simulink model "controllerSoln"  (R2018a)
settings: Solver=FixedStepAuto  StartTime=0.0  StopTime=10.0  RelTol=1e-3
PreLoadFcn:
  | initParams;
undefined symbols (not defined in the file or in its folder): DiscIntNeverNeededParam, Fc, Kd, Ki, Kp, Ts
settings Model: TunableVars=Kd,Ki,Kp  TunableVarsStorageClass=ExportedGlobal,ExportedGlobal,ExportedGlobal  TunableVarsTypeQualifier=,,  Creator=sseshadr  LastModifiedBy=scastro
settings DataIOCC: ExternalInput=testData1  LoadExternalInput=on  SaveFormat=Array
settings OptimizationCC: DefaultParameterBehavior=Inlined  EnhancedBackFolding=on  GlobalBufferReuse=off  PassReuseOutputArgsAs=Individual arguments  ZeroExternalMemoryAtStartup=off  ZeroInternalMemoryAtStartup=off  OptimizeBlockOrder=speed  DifferentSizesBufferReuse=on
settings DebuggingCC: ParameterTunabilityLossMsg=error
settings SFSimCC: MATLABDynamicMemAlloc=off
settings RTWCC: SystemTargetFile=ert.tlc  TemplateMakefile=ert_default_tmf  GenerateReport=on  IncludeHyperlinkInReport=on  LaunchReport=on  GenerateTraceInfo=on  GenerateTraceReport=on  GenerateTraceReportSl=on  GenerateTraceReportSf=on  GenerateTraceReportEml=on
settings CodeAppCC: ForceParamTrailComments=on  IgnoreCustomStorageClasses=off  OperatorAnnotations=on  SimulinkDataObjDesc=on  SFDataObjDesc=on  InsertBlockDesc=on
settings ERTTargetCC: TargetLangStandard=C99 (ISO)  GenerateSampleERTMain=on  IncludeMdlTerminateFcn=off  MatFileLogging=on  SupportComplex=off  InlinedParameterPlacement=NonHierarchical  ERTCustomFileTemplate=example_file_process.tlc

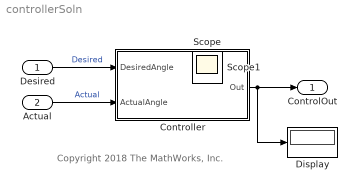
== system controllerSoln ==
  note: Copyright 2018 The MathWorks, Inc.
  Desired : Inport
  Actual : Inport  Port=2
  Controller : Subsystem
  Display : Display
  ControlOut : Outport
  Scope : Scope
  Scope1 : Scope
  wires:
  Controller/1(Out) -> Display/1, ControlOut/1
  Desired/1 -> Controller/1(DesiredAngle)  "Desired"
  Actual/1 -> Controller/2(ActualAngle)  "Actual"

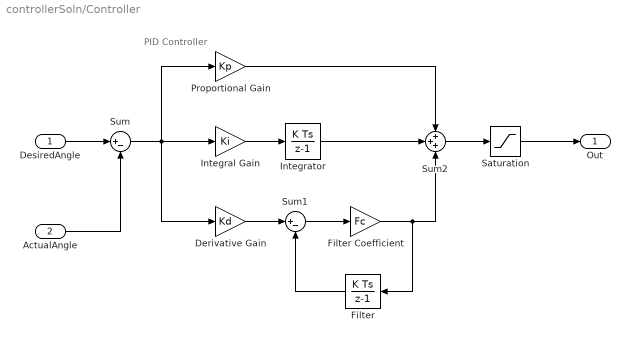
== system controllerSoln/Controller ==
  note: PID Controller
  DesiredAngle : Inport
  ActualAngle : Inport  Port=2
  Derivative Gain : Gain  Gain=Kd
  Filter : DiscreteIntegrator  DisableCoverage=on  SampleTime=Ts  ICPrevOutput=DiscIntNeverNeededParam  ICPrevScaledInput=DiscIntNeverNeededParam
  Filter Coefficient : Gain  Gain=Fc
  Integral Gain : Gain  Gain=Ki
  Integrator : DiscreteIntegrator  SampleTime=Ts  ICPrevOutput=DiscIntNeverNeededParam  ICPrevScaledInput=DiscIntNeverNeededParam
  Proportional Gain : Gain  Gain=Kp
  Saturation : Saturate  UpperLimit=5  LowerLimit=-5
  Sum : Sum  Inputs=|+-
  Sum1 : Sum  Inputs=|+-
  Sum2 : Sum  Inputs=+++
  Out : Outport
  wires:
  ActualAngle/1 -> Sum/2
  DesiredAngle/1 -> Sum/1
  Saturation/1 -> Out/1
  Sum/1 -> Derivative Gain/1, Proportional Gain/1, Integral Gain/1
  Integral Gain/1 -> Integrator/1
  Derivative Gain/1 -> Sum1/1
  Filter/1 -> Sum1/2
  Sum1/1 -> Filter Coefficient/1
  Filter Coefficient/1 -> Sum2/3, Filter/1
  Sum2/1 -> Saturation/1
  Integrator/1 -> Sum2/2
  Proportional Gain/1 -> Sum2/1
